simulink model "Series_R2015b"  (R2017a)
settings: Solver=ode4  StartTime=0  StopTime=1200  FixedStep=0.1  MaxStep=0.05  RelTol=1e-5
values from neighbouring files (symbols this model uses):
  Av = 1.725*1.490    (= 2.57025)    [Series_initiate.m]
  Cd = 0.26    [Series_initiate.m]
  Cr = 0.008    [Series_initiate.m]
  Density = (85*19.6e6 + 15*32e6)/100    (= 21460000)    [Series_initiate.m]
  EtaPE = 0.98    [Series_initiate.m]
  gr2 = 5    [Series_initiate.m]
  grav = 9.81    [Series_initiate.m]
  Jgenset = 0.1    [Series_initiate.m]
  kgenset = Jgenset/4/0.05    (= 0.5)    [Series_initiate.m]
  ksoc = Wbatt/400/Tau_charge    (= 11700)    [Series_initiate.m]
  Mv = 1325 + 250    (= 1575)    [Series_initiate.m]
  OnOffMax = SOC_batt_ref_value-eps    [Series_initiate.m]
  OnOffMin = 30    [Series_initiate.m]
  Paux = 600    [Series_initiate.m]
  Pice_max = 20E3    (= 20000)    [Series_initiate.m]
  rho_air = 1.225    [Series_initiate.m]
  rw = 0.30    (= 0.3)    [Series_initiate.m]
  SOC_batt_ref_value = 70    [Series_initiate.m]
  Tau_charge = 1    [Series_initiate.m]
  Tem1_max = 1.2*Tice_max    [Series_initiate.m]
  Tem2_max = 400+105    (= 505)    [Series_initiate.m]
  Tice_max = Pice_max/(wice_max*row/(length(EtaICE)-1))    [Series_initiate.m]
  Wbatt = 100*3600*13    (= 4680000)    [Series_initiate.m]
  wice_max = 4500*2*pi/60    (= 471.238898038)    [Series_initiate.m]
  wice_min = 800*2*pi/60    (= 83.7758040957)    [Series_initiate.m]
undefined symbols (not defined in the file or in its folder): EtaBATT, EtaEM1, EtaEM2, Pbatt, Pice_max_parallel, PtoT, sfunxy, Tlim_ice, Wice
undefined symbols (not defined in the file): EtaICE, FuelConsICE, Pem1_max, Pem2_max, Tem1, Tem2, Tice, Wem1, Wem2
settings Model: ExtModeTrigMode=oneshot  ExtModeArmWhenConnect=off  Creator=matsl  LastModifiedBy=Oskar
settings DataIOCC: SaveFormat=Array  SignalLoggingSaveFormat=ModelDataLogs  SignalLoggingName=sigsOut
settings OptimizationCC: BlockReduction=off  BooleanDataType=off  ExpressionDepthLimit=2147483647  InitFltsAndDblsToZero=on  LifeSpan=inf
settings DebuggingCC: ConsistencyChecking=warning  SaveWithParameterizedLinksMsg=none  UnderspecifiedInitializationDetection=Classic  MergeDetectMultiDrivingBlocksExec=none  SignalResolutionControl=TryResolveAllWithWarning  MultiTaskDSMMsg=warning  MultiTaskCondExecSysMsg=none  UnnecessaryDatatypeConvMsg=warning  FcnCallInpInsideContextMsg=warning  UnconnectedInputMsg=none  UnconnectedOutputMsg=none  UnconnectedLineMsg=none  AllowSymbolicDim=off  StateNameClashWarn=warning  SFUnexpectedBacktrackingDiag=warning  SFNoUnconditionalDefaultTransitionDiag=warning  SFExecutionAtInitializationDiag=none
settings HardwareCC: ProdBitPerPointer=32  ProdBitPerSizeT=32  ProdBitPerPtrDiffT=32  ProdLargestAtomicFloat=None  ProdIntDivRoundTo=Undefined  ProdEndianess=Unspecified  ProdWordSize=32  ProdHWDeviceType=32-bit Generic  TargetUnknown=on
settings ModelReferenceCC: PropagateSignalLabelsOutOfModel=off
settings GRTTargetCC: TargetLangStandard=C89/C90 (ANSI)  CombineOutputUpdateFcns=off  GRTInterface=on
settings ConfigComp: CovMetricSettings=dw  CovHtmlReporting=on  CovSaveCumulativeToWorkspaceVar=on  CovSaveSingleToWorkspaceVar=on  CovExternalEMLEnable=off

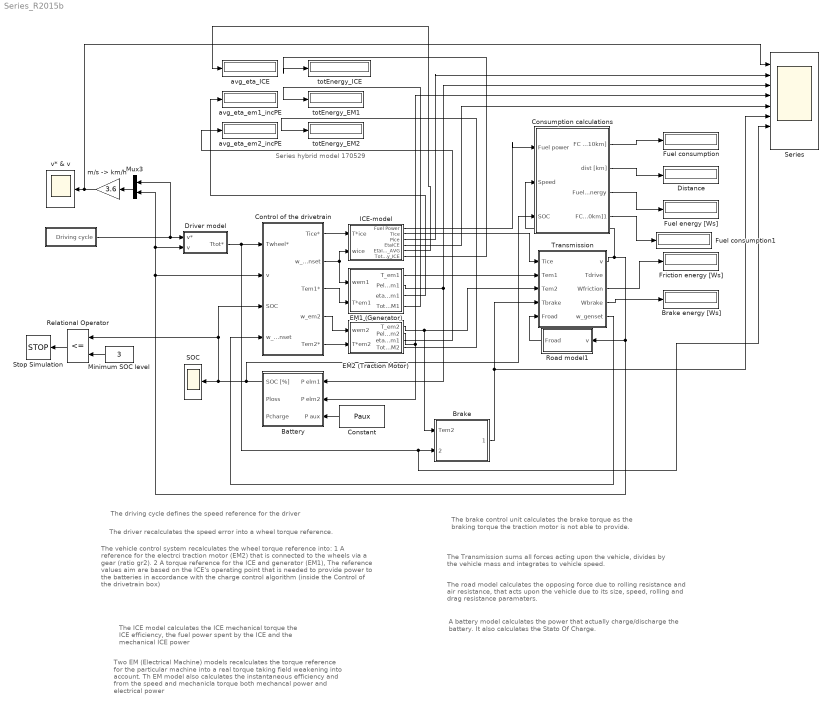
== system Series_R2015b ==
  note: Series hybrid model 170529
  note: The ICE model calculates the ICE mechanical torque
      | the ICE efficiency, the fuel power spent by the ICE
      | and the mechanical ICE power
  note: Two EM (Electrical Machine) models recalculates the
      | torque reference for the particular machine into a real
      | torque taking field weakening into account. Th EM model also
      | calculates the instantaneous efficiency and from the speed
      | and mechanicla torque both mechancal power and electrical power
  note: A battery model calculates the power that actually charge/discharge
      | the battery.
      | It also calculates the Stato Of Charge.
  note: The driving cycle defines the speed reference for the driver
  note: The brake control unit calculates the brake torque as
      | the braking torque the traction motor is not able
      | to provide.
  note: The Transmission sums all forces acting upon the vehicle, divides
      | by the vehicle mass and integrates to vehicle speed.
  note: The road model calculates the opposing force due to rolling resistance
      | and air resistance, that acts upon the vehicle due to its size, speed,
      | rolling and drag resistance paramaters.
  note: The driver recalculates the speed error into a wheel torque reference.
  note: The vehicle control system recalculates the wheel torque reference into:
      | 1	     A reference for the electrci traction motor (EM2) that is
      | connected to the wheels via a gear (ratio gr2).
      | 2	     A torque reference for the ICE and generator (EM1),
      | The reference values aim are based on the ICE's operating point that is needed
      | to provide power to the batteries in accordance with the charge control
      | algorithm (inside the Control of the drivetrain box)
  " " : Subsystem  mask{Cycle=IdealMotion}
      mask prompts: Cycle "Driving cycle"
      mask TypeOptions Cycle: nedc | us06 | IdealMotion
  Battery : Subsystem
  Brake : Subsystem
  Brake energy [Ws] : Display
  Constant : Constant  Value=Paux
  Consumption calculations : Subsystem
  Control of the drivetrain : Subsystem
  Distance : Display
  "Driver model " : Subsystem  mask{Mv=Mv, rw=rw, T_max=Tem2_max*gr2}
      mask prompts: Mv "Vehicle Mass"; rw "Wheel Radius"; T_max "Max Wheel Torque"
      mask init:
      | Ti = 3 + 7*(Mv-1000)/9000;
      | Kv=4*Mv/Ti;
  EM1 (Generator) : Subsystem
  EM2 (Traction Motor) : Subsystem
  Friction energy [Ws] : Display
  Fuel consumption : Display
  Fuel consumption1 : Display
  Fuel energy [Ws] : Display
  ICE-model : Subsystem
  Minimum SOC level : Constant  Value=3
  Mux3 : Mux  Inputs=2
  Relational Operator : RelationalOperator  Operator=<=  OutDataTypeStr=boolean  RndMeth=Nearest
  Road model1 : Subsystem
  SOC : Scope
  Series : Scope  NumInputPorts=8
  Stop Simulation : Stop
  Transmission : Subsystem
  avg_eta_ICE : Display
  avg_eta_em1_incPE : Display
  avg_eta_em2_incPE : Display
  "m/s -> km/h" : Gain  Gain=3.6  SaturateOnIntegerOverflow=on  OutDataTypeStr=Inherit: Same as input  ParamDataTypeStr=Inherit: Same as input
  totEnergy_EM1 : Display
  totEnergy_EM2 : Display
  totEnergy_ICE : Display
  v* & v : Scope
  wires:
  Constant/1 -> Battery/3(P aux)
  " "/1(Driving cycle) -> Mux3/1, "Driver model "/1(v*)
  "Driver model "/1(Ttot*) -> Series/7, Brake/2(T*wheel), Control of the drivetrain/1(Twheel*)
  Mux3/1 -> "m/s -> km/h"/1
  Transmission/1(v) -> Consumption calculations/2(Speed), Control of the drivetrain/2(v), Mux3/2, "Driver model "/2(v), Road model1/1("v ")
  ICE-model/1(Fuel Power) -> Consumption calculations/1(Fuel power)
  Transmission/3(Wfriction) -> Friction energy [Ws]/1
  Transmission/4(Wbrake) -> Brake energy [Ws]/1
  Brake/1(T_brake) -> Transmission/4(Tbrake), Series/6
  ICE-model/2(Tice) -> Transmission/1(Tice)
  EM1 (Generator)/1(T_em1) -> Transmission/2(Tem1)
  EM2 (Traction Motor)/1(T_em2) -> Brake/1(Tem2), Transmission/3(Tem2)
  Control of the drivetrain/3(Tem1*) -> EM1 (Generator)/2(T*em1)
  Control of the drivetrain/1(Tice*) -> ICE-model/1(T*ice)
  Control of the drivetrain/2("w_genset ") -> EM1 (Generator)/1(wem1), ICE-model/2(wice)
  Transmission/5(w_genset) -> Control of the drivetrain/4(w_genset)
  Control of the drivetrain/4(w_em2) -> EM2 (Traction Motor)/1(wem2)
  EM1 (Generator)/2(Pel_em1) -> Battery/1(P elm1), Series/3
  EM2 (Traction Motor)/2(Pel_em2) -> Battery/2(P elm2), Series/4
  ICE-model/3(Pice) -> Series/2
  ICE-model/4(EtaICE) -> Series/5
  Control of the drivetrain/5(Tem2*) -> EM2 (Traction Motor)/2(T*em2)
  Consumption calculations/1(FC [l/10km]) -> Fuel consumption/1
  Consumption calculations/3(FuelEnergy) -> Fuel energy [Ws]/1
  Road model1/1(Froad) -> Transmission/5(Froad)
  "m/s -> km/h"/1 -> Series/1, v* & v/1
  Consumption calculations/2(dist [km]) -> Distance/1
  Relational Operator/1 -> Stop Simulation/1
  Minimum SOC level/1 -> Relational Operator/2
  Battery/1(SOC [%]) -> Consumption calculations/3(SOC), Relational Operator/1, Control of the drivetrain/3(SOC), SOC/1
  EM1 (Generator)/3(eta_avg_em1) -> avg_eta_em1_incPE/1
  EM2 (Traction Motor)/3(eta_avg_em1) -> avg_eta_em2_incPE/1
  ICE-model/5(EtaICE_AVG) -> avg_eta_ICE/1
  EM2 (Traction Motor)/4(Total_Energy_EM2) -> totEnergy_EM2/1
  EM1 (Generator)/4(Total_Energy_EM1) -> totEnergy_EM1/1
  ICE-model/6(Total_Energy_ICE) -> totEnergy_ICE/1
  Consumption calculations/4(FC_TOT [l/10km]1) -> Fuel consumption1/1

== system Series_R2015b/  ==
  Constant : Constant  Value=Cycle
  Multiport Switch : MultiPortSwitch  SaturateOnIntegerOverflow=on  InputSameDT=on
  v-buss1 : FromWorkspace  VariableName=us06  SampleTime=.1
  v-buss2 : FromWorkspace  VariableName=IdealMotion  SampleTime=.1
  v-buss8 : FromWorkspace  VariableName=nedc  SampleTime=.1
  Driving cycle : Outport
  wires:
  v-buss8/1 -> Multiport Switch/2
  Constant/1 -> Multiport Switch/1
  v-buss1/1 -> Multiport Switch/3
  v-buss2/1 -> Multiport Switch/4
  Multiport Switch/1 -> Driving cycle/1

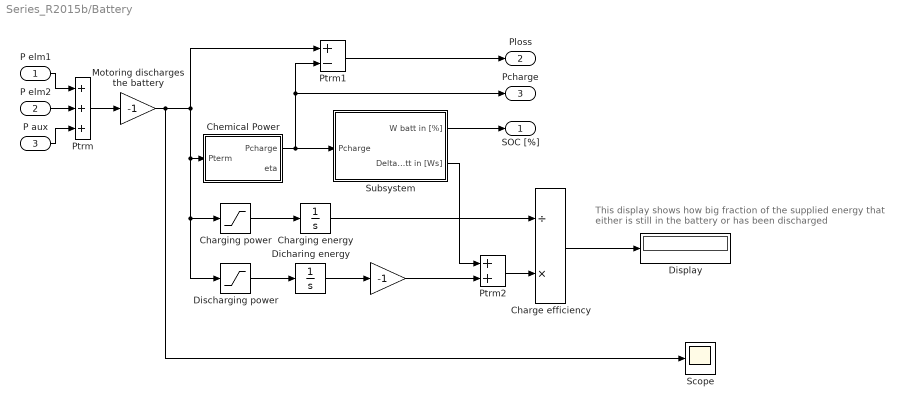
== system Series_R2015b/Battery ==
  note: This display shows how big fraction of the supplied energy
      | that either is still in the battery or has been discharged
  P elm1 : Inport
  P elm2 : Inport  Port=2
  P aux : Inport  Port=3
  " " : Gain  Gain=-1  SaturateOnIntegerOverflow=on  OutDataTypeStr=Inherit: Same as input  ParamDataTypeStr=Inherit: Same as input
  Charge efficiency : Product  Inputs=/*  SaturateOnIntegerOverflow=on  OutDataTypeStr=Inherit: Same as first input
  Charging energy : Integrator  InitialCondition=1  LimitOutput=on  LowerSaturationLimit=1
  Charging power : Saturate  UpperLimit=inf  LowerLimit=0
  Chemical Power : Subsystem
  Dicharing energy : Integrator  InitialCondition=-1  LimitOutput=on  UpperSaturationLimit=-1
  Discharging power : Saturate  UpperLimit=0  LowerLimit=-inf
  Display : Display
  Motoring discharges the battery : Gain  Gain=-1  SaturateOnIntegerOverflow=on  OutDataTypeStr=Inherit: Same as input  ParamDataTypeStr=Inherit: Same as input
  Ptrm : Sum  Inputs=+++  SaturateOnIntegerOverflow=on  InputSameDT=on  OutDataTypeStr=Inherit: Same as first input
  Ptrm1 : Sum  Inputs=+-  SaturateOnIntegerOverflow=on  InputSameDT=on  OutDataTypeStr=Inherit: Same as first input
  Ptrm2 : Sum  SaturateOnIntegerOverflow=on  InputSameDT=on  OutDataTypeStr=Inherit: Same as first input
  Scope : Scope
  Subsystem : Subsystem
  SOC [%] : Outport  InitialOutput=0
  Ploss : Outport  Port=2  InitialOutput=0
  Pcharge : Outport  Port=3  InitialOutput=0
  wires:
  P elm1/1 -> Ptrm/1
  Ptrm/1 -> Motoring discharges the battery/1
  Subsystem/1(W batt in [%]) -> SOC [%]/1
  P aux/1 -> Ptrm/3
  P elm2/1 -> Ptrm/2
  Chemical Power/1(Pcharge) -> Ptrm1/2, Pcharge/1, Subsystem/1("Pcharge ")
  Ptrm1/1 -> Ploss/1
  Motoring discharges the battery/1 -> Ptrm1/1, Charging power/1, Discharging power/1, Chemical Power/1(Pterm), Scope/1
  Charge efficiency/1 -> Display/1
  Charging power/1 -> Charging energy/1
  Discharging power/1 -> Dicharing energy/1
  Dicharing energy/1 -> " "/1
  Subsystem/2(DeltaWbatt in [Ws]) -> Ptrm2/1
  " "/1 -> Ptrm2/2
  Ptrm2/1 -> Charge efficiency/2
  Charging energy/1 -> Charge efficiency/1

== system Series_R2015b/Brake ==
  note: The mechanical brake is used when the traction motor is
      | not strong enough.
  Tem2 : Inport
  T*wheel : Inport  Port=2
  Brake : Scope  NumInputPorts=3
  Final gear : Gain  Gain=gr2  SaturateOnIntegerOverflow=on  OutDataTypeStr=Inherit: Same as input  ParamDataTypeStr=Inherit: Same as input
  Only negative brake torque : Saturate  UpperLimit=0  LowerLimit=-inf
  Sum3 : Sum  Inputs=+-  SaturateOnIntegerOverflow=on  InputSameDT=on  OutDataTypeStr=Inherit: Same as first input
  T_brake : Outport  InitialOutput=0
  wires:
  Sum3/1 -> Only negative brake torque/1
  Only negative brake torque/1 -> Brake/3, T_brake/1
  Tem2/1 -> Final gear/1
  T*wheel/1 -> Brake/1, Sum3/1
  Final gear/1 -> Brake/2, Sum3/2

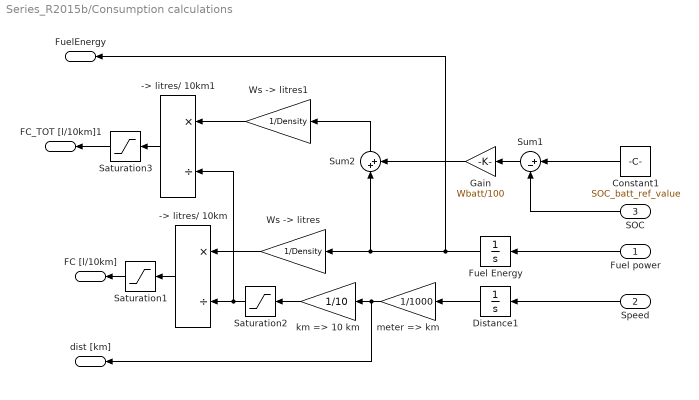
== system Series_R2015b/Consumption calculations ==
  Fuel power : Inport
  Speed : Inport  Port=2
  SOC : Inport  Port=3
  -> litres/ 10km : Product  Inputs=*/  SaturateOnIntegerOverflow=on  InputSameDT=on  OutDataTypeStr=Inherit: Same as first input
  -> litres/ 10km1 : Product  Inputs=*/  SaturateOnIntegerOverflow=on  InputSameDT=on  OutDataTypeStr=Inherit: Same as first input
  Constant1 : Constant  Value=SOC_batt_ref_value
  Distance1 : Integrator
  Fuel Energy : Integrator
  Gain : Gain  Gain=Wbatt/100
  Saturation1 : Saturate  UpperLimit=5  LowerLimit=eps
  Saturation2 : Saturate  UpperLimit=inf  LowerLimit=eps
  Saturation3 : Saturate  UpperLimit=5  LowerLimit=eps
  Sum1 : Sum  Inputs=|+-
  Sum2 : Sum  Inputs=|++
  "Ws -> litres" : Gain  Gain=1/Density  SaturateOnIntegerOverflow=on  OutDataTypeStr=Inherit: Same as input  ParamDataTypeStr=Inherit: Same as input
  "Ws -> litres1" : Gain  Gain=1/Density  SaturateOnIntegerOverflow=on  OutDataTypeStr=Inherit: Same as input  ParamDataTypeStr=Inherit: Same as input
  km => 10 km : Gain  Gain=1/10  SaturateOnIntegerOverflow=on  OutDataTypeStr=Inherit: Same as input  ParamDataTypeStr=Inherit: Same as input
  meter => km : Gain  Gain=1/1000  SaturateOnIntegerOverflow=on  OutDataTypeStr=Inherit: Same as input  ParamDataTypeStr=Inherit: Same as input
  FC [l/10km] : Outport
  dist [km] : Outport  Port=2
  FuelEnergy : Outport  Port=3
  FC_TOT [l/10km]1 : Outport  Port=4
  wires:
  Fuel power/1 -> Fuel Energy/1
  Fuel Energy/1 -> FuelEnergy/1, Sum2/1, "Ws -> litres"/1
  meter => km/1 -> dist [km]/1, km => 10 km/1
  Speed/1 -> Distance1/1
  -> litres/ 10km/1 -> Saturation1/1
  Distance1/1 -> meter => km/1
  "Ws -> litres"/1 -> -> litres/ 10km/1
  Saturation1/1 -> FC [l/10km]/1
  km => 10 km/1 -> Saturation2/1
  Saturation2/1 -> -> litres/ 10km1/2, -> litres/ 10km/2
  -> litres/ 10km1/1 -> Saturation3/1
  Saturation3/1 -> FC_TOT [l/10km]1/1
  "Ws -> litres1"/1 -> -> litres/ 10km1/1
  Constant1/1 -> Sum1/1
  Sum2/1 -> "Ws -> litres1"/1
  Gain/1 -> Sum2/2
  Sum1/1 -> Gain/1
  SOC/1 -> Sum1/2

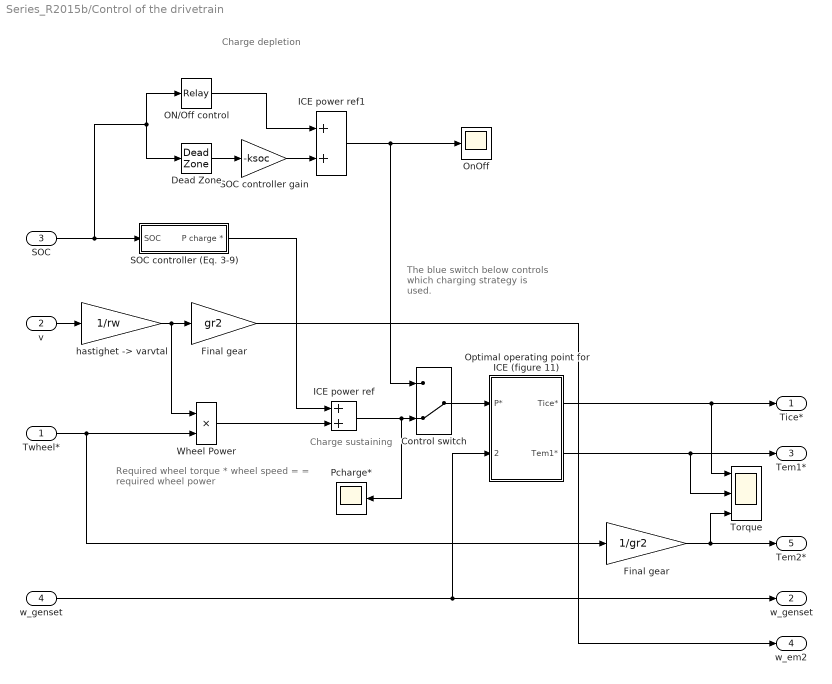
== system Series_R2015b/Control of the drivetrain ==
  note: The blue switch below
      | controls which charging
      | strategy is used.
  note: Required wheel torque * wheel speed =
      | = required wheel power
  note: Charge depletion
  note: Charge sustaining
  Twheel* : Inport
  v : Inport  Port=2
  SOC : Inport  Port=3
  w_genset : Inport  Port=4
  Control switch : ManualSwitch  CurrentSetting=0
  Dead Zone : DeadZone  LowerValue=OnOffMin  UpperValue=OnOffMax  SaturateOnIntegerOverflow=on
  Final gear : Gain  Gain=1/gr2  SaturateOnIntegerOverflow=on  OutDataTypeStr=Inherit: Same as input  ParamDataTypeStr=Inherit: Same as input
  "Final gear " : Gain  Gain=gr2  SaturateOnIntegerOverflow=on  OutDataTypeStr=Inherit: Same as input  ParamDataTypeStr=Inherit: Same as input
  ICE power ref : Sum  SaturateOnIntegerOverflow=on  InputSameDT=on  OutDataTypeStr=Inherit: Same as first input
  ICE power ref1 : Sum  SaturateOnIntegerOverflow=on  InputSameDT=on  OutDataTypeStr=Inherit: Same as first input
  ON/Off control : Relay  OnSwitchValue=OnOffMax  OffSwitchValue=OnOffMin  OnOutputValue=0  OffOutputValue=ksoc
  OnOff : Scope
  Optimal operating point for ICE (figure 11) : Subsystem
  Pcharge* : Scope
  SOC controller (Eq. 3-9) : Subsystem
  SOC controller gain : Gain  Gain=-ksoc  OutDataTypeStr=Inherit: Same as input  ParamDataTypeStr=Inherit: Same as input
  Torque : Scope  NumInputPorts=3
  Wheel Power : Product  SaturateOnIntegerOverflow=on  InputSameDT=on  OutDataTypeStr=Inherit: Same as first input
  "hastighet -> varvtal" : Gain  Gain=1/rw  SaturateOnIntegerOverflow=on  OutDataTypeStr=Inherit: Same as input  ParamDataTypeStr=Inherit: Same as input
  Tice* : Outport
  "w_genset " : Outport  Port=2
  Tem1* : Outport  Port=3
  w_em2 : Outport  Port=4
  Tem2* : Outport  Port=5
  wires:
  "hastighet -> varvtal"/1 -> Wheel Power/1, "Final gear "/1
  Twheel*/1 -> Wheel Power/2, Final gear/1
  v/1 -> "hastighet -> varvtal"/1
  SOC/1 -> SOC controller (Eq. 3-9)/1(SOC), Dead Zone/1, ON/Off control/1
  Wheel Power/1 -> ICE power ref/2
  SOC controller (Eq. 3-9)/1(P charge *) -> ICE power ref/1
  Optimal operating point for ICE (figure 11)/2(Tem1*) -> Tem1*/1, Torque/2
  Optimal operating point for ICE (figure 11)/1(Tice*) -> Tice*/1, Torque/1
  w_genset/1 -> Optimal operating point for ICE (figure 11)/2(w_genset), "w_genset "/1
  Final gear/1 -> Tem2*/1, Torque/3
  "Final gear "/1 -> w_em2/1
  Dead Zone/1 -> SOC controller gain/1
  ON/Off control/1 -> ICE power ref1/1
  SOC controller gain/1 -> ICE power ref1/2
  Control switch/1 -> Optimal operating point for ICE (figure 11)/1(P*)
  ICE power ref1/1 -> OnOff/1, Control switch/1
  ICE power ref/1 -> Control switch/2, Pcharge*/1

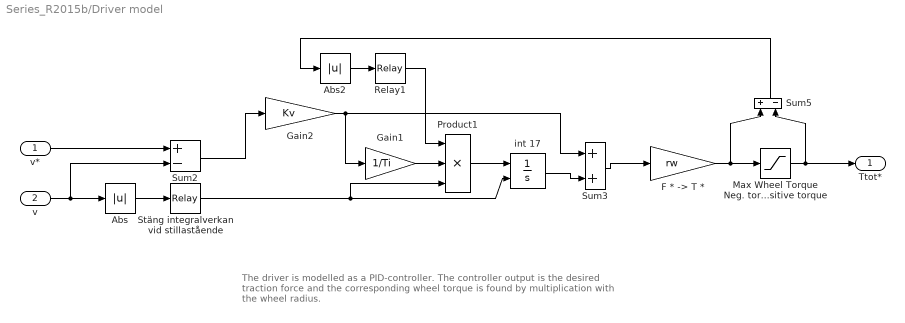
== system Series_R2015b/Driver model  ==
  note: The driver is modelled as a PID-controller.
      | The controller output is the desired traction force and the
      | corresponding wheel torque is found by multiplication with the wheel radius.
  v* : Inport
  v : Inport  Port=2
  Abs : Abs  SaturateOnIntegerOverflow=on
  Abs2 : Abs  SaturateOnIntegerOverflow=on
  "F * -> T *" : Gain  Gain=rw  SaturateOnIntegerOverflow=on  OutDataTypeStr=Inherit: Same as input  ParamDataTypeStr=Inherit: Same as input
  Gain1 : Gain  Gain=1/Ti  SaturateOnIntegerOverflow=on  OutDataTypeStr=Inherit: Same as input  ParamDataTypeStr=Inherit: Same as input
  Gain2 : Gain  Gain=Kv  SaturateOnIntegerOverflow=on  OutDataTypeStr=Inherit: Same as input  ParamDataTypeStr=Inherit: Same as input
  Max Wheel Torque Neg. torque can be 5 times positive torque : Saturate  UpperLimit=T_max  LowerLimit=-T_max*5
  Product1 : Product  Inputs=3  SaturateOnIntegerOverflow=on  InputSameDT=on  OutDataTypeStr=Inherit: Same as first input
  Relay1 : Relay  OnOutputValue=0  OffOutputValue=1
  Stäng integralverkan vid stillastående : Relay  OnSwitchValue=0.3  OffSwitchValue=0.3-eps
  Sum2 : Sum  Inputs=+-  SaturateOnIntegerOverflow=on  InputSameDT=on  OutDataTypeStr=Inherit: Same as first input
  Sum3 : Sum  SaturateOnIntegerOverflow=on  InputSameDT=on  OutDataTypeStr=Inherit: Same as first input
  Sum5 : Sum  Inputs=+-  SaturateOnIntegerOverflow=on  InputSameDT=on  OutDataTypeStr=Inherit: Same as first input
  int 17 : Integrator  ExternalReset=falling  LimitOutput=on  UpperSaturationLimit=1000  LowerSaturationLimit=-10000
  Ttot* : Outport  InitialOutput=0
  wires:
  v/1 -> Sum2/2, Abs/1
  v*/1 -> Sum2/1
  Sum2/1 -> Gain2/1
  Stäng integralverkan vid stillastående/1 -> int 17/2, Product1/3
  Gain2/1 -> Sum3/1, Gain1/1
  "F * -> T *"/1 -> Max Wheel Torque Neg. torque can be 5 times positive torque/1, Sum5/1
  int 17/1 -> Sum3/2
  Sum3/1 -> "F * -> T *"/1
  Product1/1 -> int 17/1
  Abs/1 -> Stäng integralverkan vid stillastående/1
  Gain1/1 -> Product1/2
  Abs2/1 -> Relay1/1
  Relay1/1 -> Product1/1
  Sum5/1 -> Abs2/1
  Max Wheel Torque Neg. torque can be 5 times positive torque/1 -> Ttot*/1, Sum5/2

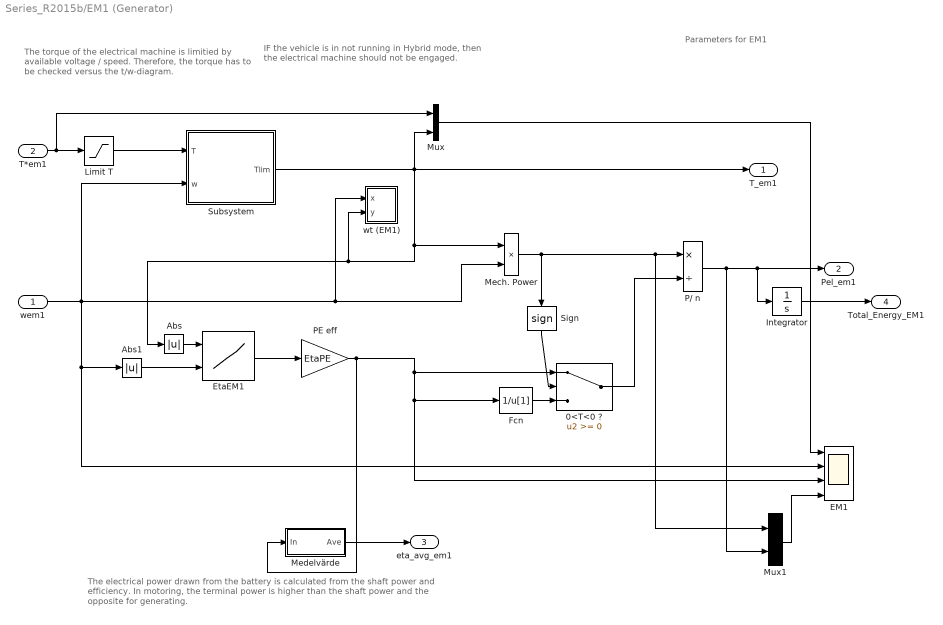
== system Series_R2015b/EM1 (Generator) ==
  note: The torque of the electrical machine is
      | limitied by available voltage / speed. Therefore, the
      | torque has to be checked versus the t/w-diagram.
  note: IF the vehicle is in not running in Hybrid mode, then
      | the electrical machine should not be engaged.
  note: The electrical power drawn from the battery is calculated from the shaft power and
      | efficiency. In motoring, the terminal power is higher than the shaft power and
      | the opposite for  generating.
  note: Parameters for EM1
  wem1 : Inport
  T*em1 : Inport  Port=2
  0<T<0 ? : Switch  SaturateOnIntegerOverflow=on  InputSameDT=on
  Abs : Abs  SaturateOnIntegerOverflow=on
  Abs1 : Abs  SaturateOnIntegerOverflow=on
  EM1 : Scope  NumInputPorts=4
  EtaEM1 : Lookup2D  RowIndex=Tem1  ColumnIndex=Wem1  Table=EtaEM1  LookUpMeth=Interpolation-Use End Values  SaturateOnIntegerOverflow=on
  Fcn : Fcn  Expr=1/u[1]
  Integrator : Integrator
  Limit T : Saturate  UpperLimit=Tem1_max  LowerLimit=-Tem1_max
  Mech. Power : Product  SaturateOnIntegerOverflow=on  OutDataTypeStr=Inherit: Same as first input
  Medelvärde : Subsystem
  Mux : Mux  Inputs=2
  Mux1 : Mux  Inputs=2
  P/ n : Product  Inputs=*/  SaturateOnIntegerOverflow=on  InputSameDT=on  OutDataTypeStr=Inherit: Same as first input
  PE eff : Gain  Gain=EtaPE  SaturateOnIntegerOverflow=on  OutDataTypeStr=Inherit: Same as input  ParamDataTypeStr=Inherit: Same as input
  Sign : Signum
  Subsystem : Subsystem  mask{Tmax=Tem1_max, Pmax=Pem1_max}
      mask prompts: Tmax "Max Torque"; Pmax "Max Power"
      mask Display:
      | plot(-120,-120,120,120)
      | plot([-110 110],[0 0],[0 0],[-110 110])
      | plot([-20 20],[90 90],[-20 20],[-90 -90])
      | 
      | plot([-100 :-20],-90*20./[-100:-20])
      | plot([-100 :-20],90*20./[-100:-20])
      | plot([20:100],-90*20./[20:100])
      | plot([20:100],90*20./[20:100])
  wt (EM1) : Subsystem  AncestorBlock=simulink/Sinks/XY Graph  LoadFcn=sfunxy([],[],[],'LoadBlock')  StartFcn=sfunxy([],[],[],'Start')  StopFcn=sfunxy([],[],[],'Stop')  TreatAsAtomicUnit=on  SimViewingDevice=on  mask(XY scope.){xmin=-max(Wem1)*1.2, xmax=max(Wem1)*1.2, ymin=-max(Tem1)*1.2, ymax=max(Tem1)*1.2, st=1}
      mask prompts: xmin "x-min:"; xmax "x-max:"; ymin "y-min:"; ymax "y-max:"; st "Sample time:"
      mask help: Plots second input (Y) against first input (X) at each time step to create an X-Y plot. Ignores data outside the ranges specified by x-min, x-max, y-min, y-max.
      settings: CopyFcn=sfunxy([],[],[],'CopyBlock')  DeleteFcn=sfunxy([],[],[],'DeleteBlock')  NameChangeFcn=sfunxy([],[],[],'NameChange')
      mask Help: This block can be used to explore limit cycles. Look at the m-file sfunxy.m to see how it works.
      mask Display: plot([.05 .95 .95 .05 .05],[.45 .45 .95 .95 .45], 0.5+cos(0:0.1:2*pi)*0.3,0.7+sin(0:0.1:2*pi)*0.2)
  T_em1 : Outport  InitialOutput=0
  Pel_em1 : Outport  Port=2  InitialOutput=0
  eta_avg_em1 : Outport  Port=3  InitialOutput=0
  Total_Energy_EM1 : Outport  Port=4  InitialOutput=0
  wires:
  EtaEM1/1 -> PE eff/1
  Subsystem/1(Tlim) -> Mech. Power/1, wt (EM1)/2(y), Abs/1, T_em1/1, Mux/2
  Sign/1 -> 0<T<0 ?/2
  P/ n/1 -> Mux1/2, Integrator/1, Pel_em1/1
  T*em1/1 -> Limit T/1, Mux/1
  Fcn/1 -> 0<T<0 ?/3
  0<T<0 ?/1 -> P/ n/2
  Abs/1 -> EtaEM1/1
  Limit T/1 -> Subsystem/1(T)
  wem1/1 -> EM1/2, Abs1/1, wt (EM1)/1(x), Mech. Power/2, Subsystem/2(w)
  PE eff/1 -> Medelvärde/1(In), EM1/3, Fcn/1, 0<T<0 ?/1
  Mux/1 -> EM1/1
  Mux1/1 -> EM1/4
  Mech. Power/1 -> Sign/1, Mux1/1, P/ n/1
  Abs1/1 -> EtaEM1/2
  Medelvärde/1(Ave) -> eta_avg_em1/1
  Integrator/1 -> Total_Energy_EM1/1

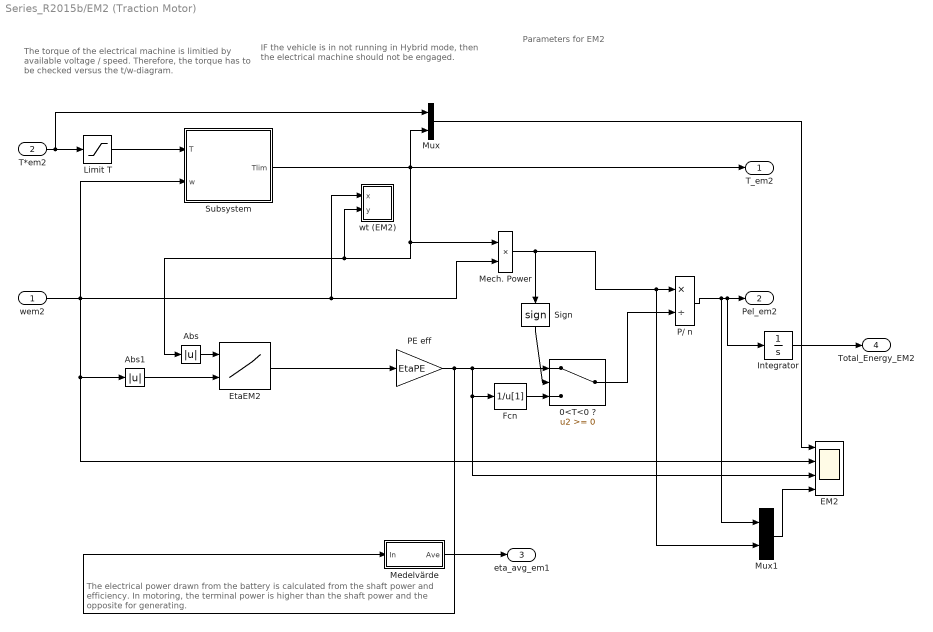
== system Series_R2015b/EM2 (Traction Motor) ==
  note: The torque of the electrical machine is
      | limitied by available voltage / speed. Therefore, the
      | torque has to be checked versus the t/w-diagram.
  note: IF the vehicle is in not running in Hybrid mode, then
      | the electrical machine should not be engaged.
  note: The electrical power drawn from the battery is calculated from the shaft power and
      | efficiency. In motoring, the terminal power is higher than the shaft power and
      | the opposite for  generating.
  note: Parameters for EM2
  wem2 : Inport
  T*em2 : Inport  Port=2
  0<T<0 ? : Switch  SaturateOnIntegerOverflow=on  InputSameDT=on
  Abs : Abs  SaturateOnIntegerOverflow=on
  Abs1 : Abs  SaturateOnIntegerOverflow=on
  EM2 : Scope  NumInputPorts=4
  EtaEM2 : Lookup2D  RowIndex=Tem2  ColumnIndex=Wem2  Table=EtaEM2  LookUpMeth=Interpolation-Use End Values  SaturateOnIntegerOverflow=on
  Fcn : Fcn  Expr=1/u[1]
  Integrator : Integrator
  Limit T : Saturate  UpperLimit=Tem2_max  LowerLimit=-Tem2_max
  Mech. Power : Product  SaturateOnIntegerOverflow=on  OutDataTypeStr=Inherit: Same as first input
  Medelvärde : Subsystem
  Mux : Mux  Inputs=2
  Mux1 : Mux  Inputs=2
  P/ n : Product  Inputs=*/  SaturateOnIntegerOverflow=on  InputSameDT=on  OutDataTypeStr=Inherit: Same as first input
  PE eff : Gain  Gain=EtaPE  SaturateOnIntegerOverflow=on  OutDataTypeStr=Inherit: Same as input  ParamDataTypeStr=Inherit: Same as input
  Sign : Signum
  Subsystem : Subsystem  mask{Tmax=Tem2_max, Pmax=Pem2_max}
      mask prompts: Tmax "Max Torque"; Pmax "Max Power"
      mask Display:
      | plot(-120,-120,120,120)
      | plot([-110 110],[0 0],[0 0],[-110 110])
      | plot([-20 20],[90 90],[-20 20],[-90 -90])
      | 
      | plot([-100 :-20],-90*20./[-100:-20])
      | plot([-100 :-20],90*20./[-100:-20])
      | plot([20:100],-90*20./[20:100])
      | plot([20:100],90*20./[20:100])
  wt (EM2) : Subsystem  AncestorBlock=simulink/Sinks/XY Graph  LoadFcn=sfunxy([],[],[],'LoadBlock')  StartFcn=sfunxy([],[],[],'Start')  StopFcn=sfunxy([],[],[],'Stop')  TreatAsAtomicUnit=on  SimViewingDevice=on  mask(XY scope.){xmin=-max(Wem2)*1.2, xmax=max(Wem2)*1.2, ymin=-max(Tem2)*1.2, ymax=max(Tem2)*1.2, st=1}
      mask prompts: xmin "x-min:"; xmax "x-max:"; ymin "y-min:"; ymax "y-max:"; st "Sample time:"
      mask help: Plots second input (Y) against first input (X) at each time step to create an X-Y plot. Ignores data outside the ranges specified by x-min, x-max, y-min, y-max.
      settings: CopyFcn=sfunxy([],[],[],'CopyBlock')  DeleteFcn=sfunxy([],[],[],'DeleteBlock')  NameChangeFcn=sfunxy([],[],[],'NameChange')
      mask Help: This block can be used to explore limit cycles. Look at the m-file sfunxy.m to see how it works.
      mask Display: plot([.05 .95 .95 .05 .05],[.45 .45 .95 .95 .45], 0.5+cos(0:0.1:2*pi)*0.3,0.7+sin(0:0.1:2*pi)*0.2)
  T_em2 : Outport  InitialOutput=0
  Pel_em2 : Outport  Port=2  InitialOutput=0
  eta_avg_em1 : Outport  Port=3  InitialOutput=0
  Total_Energy_EM2 : Outport  Port=4  InitialOutput=0
  wires:
  EtaEM2/1 -> PE eff/1
  Subsystem/1(Tlim) -> Mech. Power/1, wt (EM2)/2(y), Abs/1, T_em2/1, Mux/2
  Sign/1 -> 0<T<0 ?/2
  P/ n/1 -> Mux1/1, Integrator/1, Pel_em2/1
  T*em2/1 -> Limit T/1, Mux/1
  Fcn/1 -> 0<T<0 ?/3
  0<T<0 ?/1 -> P/ n/2
  Abs/1 -> EtaEM2/1
  Limit T/1 -> Subsystem/1(T)
  wem2/1 -> EM2/2, Abs1/1, wt (EM2)/1(x), Mech. Power/2, Subsystem/2(w)
  Mux/1 -> EM2/1
  Mux1/1 -> EM2/4
  Mech. Power/1 -> Sign/1, Mux1/2, P/ n/1
  Abs1/1 -> EtaEM2/2
  PE eff/1 -> Medelvärde/1(In), EM2/3, Fcn/1, 0<T<0 ?/1
  Medelvärde/1(Ave) -> eta_avg_em1/1
  Integrator/1 -> Total_Energy_EM2/1

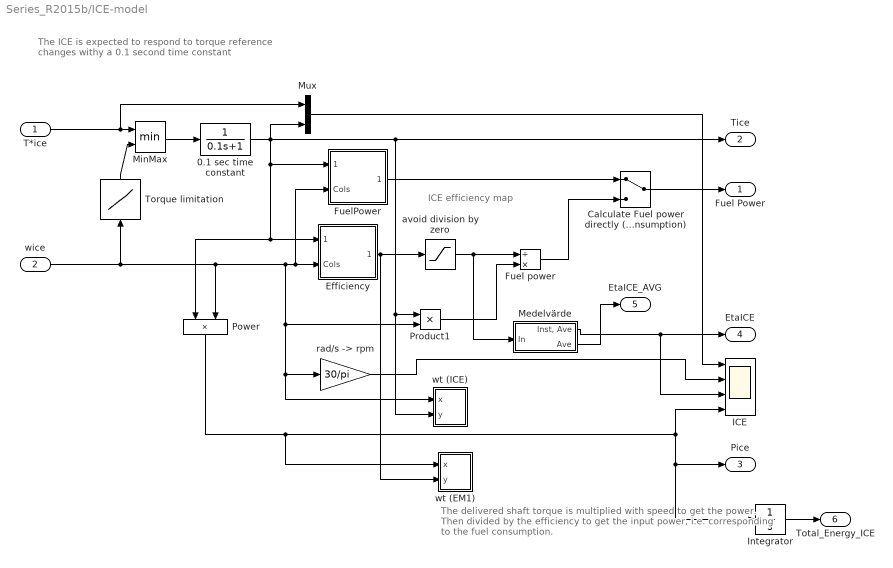
== system Series_R2015b/ICE-model ==
  note: The ICE is expected to respond to torque reference
      | changes withy a 0.1 second
      | time constant
  note: ICE efficiency map
  note: The delivered shaft torque is multiplied with speed to get the power.
      | Then divided by the efficiency to get the input power, i.e.
      | corresponding to the fuel consumption.
  T*ice : Inport
  wice : Inport  Port=2
  0.1 sec time constant : TransferFcn  Denominator=[0.1 1]
  Calculate Fuel power directly (w/o idle consumption) : ManualSwitch
  Efficiency : Subsystem  mask(Lookup Table (2-D)){x=Tice, y=Wice, t=EtaICE}
      mask prompts: x "Row:"; y "Column:"; t "Table:"
      mask help: Performs 2-D linear interpolation of input values using the specified input/output table. Extrapolation is performed outside the table boundaries. The first dimension corresponds to the top (or left) input port.
      mask init:
      | [r,c]=size(t);
      | xt=reshape(x,prod(size(x)),1);
      | xi=xt(:,ones(1,c));
      | minx=min(x); maxx=max(x);
      | mint=min(min(t)); maxt=max(max(t));
      mask Display: plot(double(xi),double(t),double([minx maxx]),double([mint mint]),double([minx minx]),double([mint maxt]))
  Fuel power : Product  Inputs=/*  SaturateOnIntegerOverflow=on  InputSameDT=on  OutDataTypeStr=Inherit: Same as first input
  FuelPower : Subsystem  mask(Lookup Table (2-D)){x=Tice, y=Wice, t=FuelConsICE}
      mask prompts: x "Row:"; y "Column:"; t "Table:"
      mask help: Performs 2-D linear interpolation of input values using the specified input/output table. Extrapolation is performed outside the table boundaries. The first dimension corresponds to the top (or left) input port.
      mask init:
      | [r,c]=size(t);
      | xt=reshape(x,prod(size(x)),1);
      | xi=xt(:,ones(1,c));
      | minx=min(x); maxx=max(x);
      | mint=min(min(t)); maxt=max(max(t));
      mask Display: plot(double(xi),double(t),double([minx maxx]),double([mint mint]),double([minx minx]),double([mint maxt]))
  ICE : Scope  NumInputPorts=4
  Integrator : Integrator
  Medelvärde : Subsystem
  MinMax : MinMax  Inputs=2  SaturateOnIntegerOverflow=on  InputSameDT=on
  Mux : Mux  Inputs=2
  Power : Product  SaturateOnIntegerOverflow=on  OutDataTypeStr=Inherit: Same as first input
  Product1 : Product  SaturateOnIntegerOverflow=on  InputSameDT=on  OutDataTypeStr=Inherit: Same as first input
  Torque limitation : Lookup  InputValues=Wice  Table=Tlim_ice  SaturateOnIntegerOverflow=on
  avoid division by zero : Saturate  UpperLimit=inf  LowerLimit=0.02
  "rad/s -> rpm" : Gain  Gain=30/pi  SaturateOnIntegerOverflow=on  OutDataTypeStr=Inherit: Same as input  ParamDataTypeStr=Inherit: Same as input
  wt (EM1) : Subsystem  AncestorBlock=simulink/Sinks/XY Graph  LoadFcn=sfunxy([],[],[],'LoadBlock')  StartFcn=sfunxy([],[],[],'Start')  StopFcn=sfunxy([],[],[],'Stop')  TreatAsAtomicUnit=on  SimViewingDevice=on  mask(XY scope.){xmin=0, xmax=Pice_max, ymin=0, ymax=1, st=1}
      mask prompts: xmin "x-min:"; xmax "x-max:"; ymin "y-min:"; ymax "y-max:"; st "Sample time:"
      mask help: Plots second input (Y) against first input (X) at each time step to create an X-Y plot. Ignores data outside the ranges specified by x-min, x-max, y-min, y-max.
      settings: CopyFcn=sfunxy([],[],[],'CopyBlock')  DeleteFcn=sfunxy([],[],[],'DeleteBlock')  NameChangeFcn=sfunxy([],[],[],'NameChange')
      mask Help: This block can be used to explore limit cycles. Look at the m-file sfunxy.m to see how it works.
      mask Display: plot([.05 .95 .95 .05 .05],[.45 .45 .95 .95 .45], 0.5+cos(0:0.1:2*pi)*0.3,0.7+sin(0:0.1:2*pi)*0.2)
  wt (ICE) : Subsystem  AncestorBlock=simulink/Sinks/XY Graph  LoadFcn=sfunxy([],[],[],'LoadBlock')  StartFcn=sfunxy([],[],[],'Start')  StopFcn=sfunxy([],[],[],'Stop')  TreatAsAtomicUnit=on  SimViewingDevice=on  mask(XY scope.){xmin=0, xmax=max(Wice)*1.2, ymin=-max(Tice)*0.2, ymax=max(Tice)*1.2, st=1}
      mask prompts: xmin "x-min:"; xmax "x-max:"; ymin "y-min:"; ymax "y-max:"; st "Sample time:"
      mask help: Plots second input (Y) against first input (X) at each time step to create an X-Y plot. Ignores data outside the ranges specified by x-min, x-max, y-min, y-max.
      settings: CopyFcn=sfunxy([],[],[],'CopyBlock')  DeleteFcn=sfunxy([],[],[],'DeleteBlock')  NameChangeFcn=sfunxy([],[],[],'NameChange')
      mask Help: This block can be used to explore limit cycles. Look at the m-file sfunxy.m to see how it works.
      mask Display: plot([.05 .95 .95 .05 .05],[.45 .45 .95 .95 .45], 0.5+cos(0:0.1:2*pi)*0.3,0.7+sin(0:0.1:2*pi)*0.2)
  Fuel Power : Outport  InitialOutput=0
  Tice : Outport  Port=2  InitialOutput=0
  Pice : Outport  Port=3  InitialOutput=0
  EtaICE : Outport  Port=4  InitialOutput=0
  EtaICE_AVG : Outport  Port=5  InitialOutput=0
  Total_Energy_ICE : Outport  Port=6  InitialOutput=0
  wires:
  Product1/1 -> Fuel power/2
  Efficiency/1(Out1) -> wt (EM1)/2(y), avoid division by zero/1
  "rad/s -> rpm"/1 -> ICE/2
  Medelvärde/1("Inst, Ave") -> ICE/3, EtaICE/1
  T*ice/1 -> Mux/1, MinMax/1
  Torque limitation/1 -> MinMax/2
  MinMax/1 -> 0.1 sec time constant/1
  Mux/1 -> ICE/1
  Power/1 -> wt (EM1)/1(x), ICE/4, Integrator/1, Pice/1
  avoid division by zero/1 -> Medelvärde/1(In), Fuel power/1
  wice/1 -> Torque limitation/1, Product1/2, wt (ICE)/1(x), "rad/s -> rpm"/1, FuelPower/2(Cols), Efficiency/2(Cols), Power/2
  0.1 sec time constant/1 -> wt (ICE)/2(y), Product1/1, Tice/1, Mux/2, FuelPower/1(Rows), Efficiency/1(Rows), Power/1
  FuelPower/1(Out1) -> Calculate Fuel power directly (w/o idle consumption)/1
  Fuel power/1 -> Calculate Fuel power directly (w/o idle consumption)/2
  Calculate Fuel power directly (w/o idle consumption)/1 -> Fuel Power/1
  Medelvärde/2(Ave) -> EtaICE_AVG/1
  Integrator/1 -> Total_Energy_ICE/1

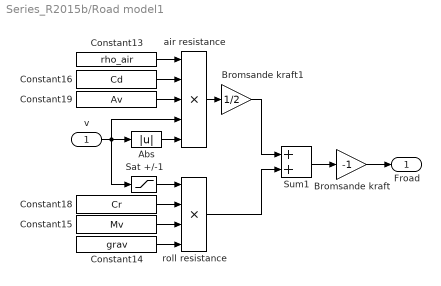
== system Series_R2015b/Road model1 ==
  "v " : Inport
  Abs : Abs  SaturateOnIntegerOverflow=on
  Bromsande kraft : Gain  Gain=-1  SaturateOnIntegerOverflow=on  OutDataTypeStr=Inherit: Same as input  ParamDataTypeStr=Inherit: Same as input
  Bromsande kraft1 : Gain  Gain=1/2  SaturateOnIntegerOverflow=on  OutDataTypeStr=Inherit: Same as input  ParamDataTypeStr=Inherit: Same as input
  Constant13 : Constant  Value=rho_air
  Constant14 : Constant  Value=grav
  Constant15 : Constant  Value=Mv
  Constant16 : Constant  Value=Cd
  Constant18 : Constant  Value=Cr
  Constant19 : Constant  Value=Av
  Sat +/-1 : Saturate  UpperLimit=1  LowerLimit=-1
  Sum1 : Sum  SaturateOnIntegerOverflow=on  InputSameDT=on  OutDataTypeStr=Inherit: Same as first input
  air resistance : Product  Inputs=5  SaturateOnIntegerOverflow=on  InputSameDT=on  OutDataTypeStr=Inherit: Same as first input
  roll resistance : Product  Inputs=4  SaturateOnIntegerOverflow=on  InputSameDT=on  OutDataTypeStr=Inherit: Same as first input
  Froad : Outport  InitialOutput=0
  wires:
  air resistance/1 -> Bromsande kraft1/1
  Bromsande kraft/1 -> Froad/1
  Bromsande kraft1/1 -> Sum1/1
  roll resistance/1 -> Sum1/2
  Sum1/1 -> Bromsande kraft/1
  Constant13/1 -> air resistance/1
  Constant16/1 -> air resistance/2
  Constant19/1 -> air resistance/3
  "v "/1 -> air resistance/4, Sat +/-1/1, Abs/1
  Constant18/1 -> roll resistance/2
  Constant15/1 -> roll resistance/3
  Constant14/1 -> roll resistance/4
  Sat +/-1/1 -> roll resistance/1
  Abs/1 -> air resistance/5

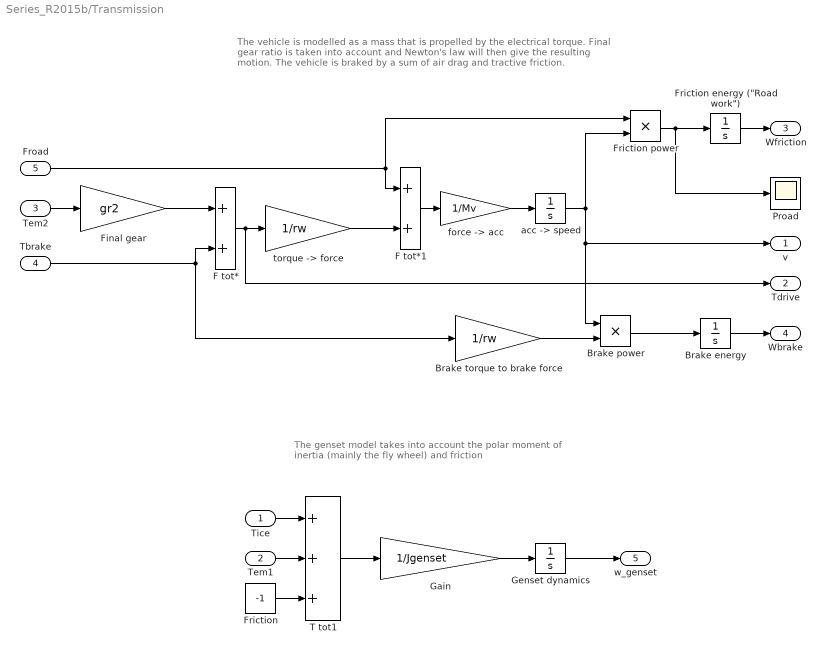
== system Series_R2015b/Transmission ==
  note: The vehicle is modelled as a mass that is propelled by the electrical torque.
      | Final gear ratio is taken into account and Newton's law will then
      | give the resulting motion.
      | The vehicle is braked by a sum of air drag and tractive friction.
  note: The genset model takes into account the polar moment
      | of inertia (mainly the fly wheel) and friction
  Tice : Inport
  Tem1 : Inport  Port=2
  Tem2 : Inport  Port=3
  Tbrake : Inport  Port=4
  Froad : Inport  Port=5
  Brake energy : Integrator
  Brake power : Product  SaturateOnIntegerOverflow=on  InputSameDT=on  OutDataTypeStr=Inherit: Same as first input
  Brake torque to brake force : Gain  Gain=1/rw  SaturateOnIntegerOverflow=on  OutDataTypeStr=Inherit: Same as input  ParamDataTypeStr=Inherit: Same as input
  F tot* : Sum  SaturateOnIntegerOverflow=on  InputSameDT=on  OutDataTypeStr=Inherit: Same as first input
  F tot*1 : Sum  SaturateOnIntegerOverflow=on  InputSameDT=on  OutDataTypeStr=Inherit: Same as first input
  Final gear : Gain  Gain=gr2  SaturateOnIntegerOverflow=on  OutDataTypeStr=Inherit: Same as input  ParamDataTypeStr=Inherit: Same as input
  Friction : Constant  Value=-1
  "Friction energy (\"Road work\")" : Integrator
  Friction power : Product  SaturateOnIntegerOverflow=on  InputSameDT=on  OutDataTypeStr=Inherit: Same as first input
  Gain : Gain  Gain=1/Jgenset  SaturateOnIntegerOverflow=on  OutDataTypeStr=Inherit: Same as input  ParamDataTypeStr=Inherit: Same as input
  Genset dynamics : Integrator
  Proad : Scope
  T tot1 : Sum  Inputs=+++  SaturateOnIntegerOverflow=on  InputSameDT=on  OutDataTypeStr=Inherit: Same as first input
  "acc -> speed" : Integrator
  "force -> acc" : Gain  Gain=1/Mv  SaturateOnIntegerOverflow=on  OutDataTypeStr=Inherit: Same as input  ParamDataTypeStr=Inherit: Same as input
  "torque -> force" : Gain  Gain=1/rw  SaturateOnIntegerOverflow=on  OutDataTypeStr=Inherit: Same as input  ParamDataTypeStr=Inherit: Same as input
  v : Outport  InitialOutput=0
  Tdrive : Outport  Port=2  InitialOutput=0
  Wfriction : Outport  Port=3  InitialOutput=0
  Wbrake : Outport  Port=4  InitialOutput=0
  w_genset : Outport  Port=5  InitialOutput=0
  wires:
  "force -> acc"/1 -> "acc -> speed"/1
  Tem2/1 -> Final gear/1
  "acc -> speed"/1 -> Brake power/1, v/1, Friction power/2
  F tot*/1 -> "torque -> force"/1, Tdrive/1
  Tbrake/1 -> F tot*/2, Brake torque to brake force/1
  "torque -> force"/1 -> F tot*1/2
  F tot*1/1 -> "force -> acc"/1
  Froad/1 -> Friction power/1, F tot*1/1
  Brake torque to brake force/1 -> Brake power/2
  Brake power/1 -> Brake energy/1
  Friction power/1 -> "Friction energy (\"Road work\")"/1, Proad/1
  "Friction energy (\"Road work\")"/1 -> Wfriction/1
  Brake energy/1 -> Wbrake/1
  Genset dynamics/1 -> w_genset/1
  Tice/1 -> T tot1/1
  Tem1/1 -> T tot1/2
  T tot1/1 -> Gain/1
  Gain/1 -> Genset dynamics/1
  Friction/1 -> T tot1/3
  Final gear/1 -> F tot*/1

== system Series_R2015b/Battery/Chemical Power ==
  Pterm : Inport
  Look-Up Table : Lookup  InputValues=Pbatt  Table=EtaBATT  SaturateOnIntegerOverflow=on
  P/ n : Product  Inputs=**  SaturateOnIntegerOverflow=on  InputSameDT=on  OutDataTypeStr=Inherit: Same as first input
  Saturation : Saturate  UpperLimit=max(Pbatt)  LowerLimit=min(Pbatt)
  Pcharge : Outport  InitialOutput=0
  eta : Outport  Port=2  InitialOutput=0
  wires:
  Pterm/1 -> P/ n/1, Saturation/1
  Saturation/1 -> Look-Up Table/1
  P/ n/1 -> Pcharge/1
  Look-Up Table/1 -> P/ n/2, eta/1

== system Series_R2015b/Battery/Subsystem ==
  "Pcharge " : Inport
  Constant : Constant  Value=SOC_batt_ref_value/100*Wbatt
  Gain3 : Gain  Gain=100/Wbatt  SaturateOnIntegerOverflow=on  OutDataTypeStr=Inherit: Same as input  ParamDataTypeStr=Inherit: Same as input
  Ptrm1 : Sum  Inputs=+-  SaturateOnIntegerOverflow=on  InputSameDT=on  OutDataTypeStr=Inherit: Same as first input
  W batt starts at SOC_batt_ref_value : Integrator  InitialCondition=SOC_batt_ref_value/100*Wbatt  LimitOutput=on  LowerSaturationLimit=0
  W batt in [%] : Outport
  DeltaWbatt in [Ws] : Outport  Port=2
  wires:
  W batt starts at SOC_batt_ref_value/1 -> Gain3/1, Ptrm1/1
  Gain3/1 -> W batt in [%]/1
  Constant/1 -> Ptrm1/2
  Ptrm1/1 -> DeltaWbatt in [Ws]/1
  "Pcharge "/1 -> W batt starts at SOC_batt_ref_value/1

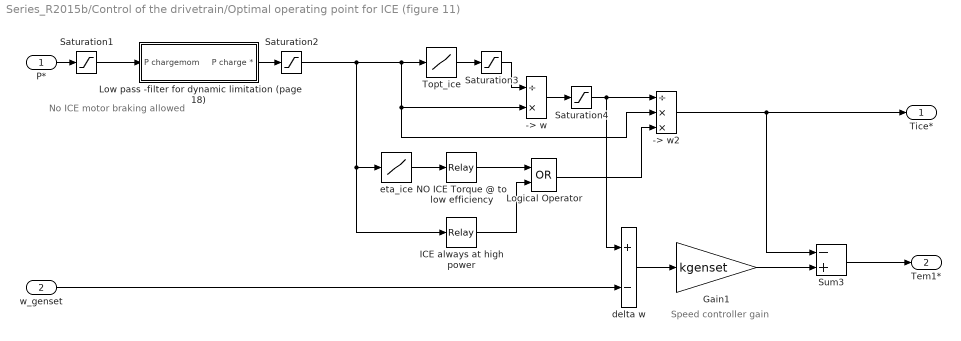
== system Series_R2015b/Control of the drivetrain/Optimal operating point for ICE (figure 11) ==
  note: No ICE motor
      | braking allowed
  note: Speed controller gain
  P* : Inport
  w_genset : Inport  Port=2
  -> w : Product  Inputs=/*  SaturateOnIntegerOverflow=on  InputSameDT=on  OutDataTypeStr=Inherit: Same as first input
  -> w2 : Product  Inputs=/**  SaturateOnIntegerOverflow=on  InputSameDT=on  OutDataTypeStr=Inherit: Same as first input
  Gain1 : Gain  Gain=kgenset  SaturateOnIntegerOverflow=on  OutDataTypeStr=Inherit: Same as input  ParamDataTypeStr=Inherit: Same as input
  ICE always at high power : Relay  OnSwitchValue=Pice_max/1.8*1.1  OffSwitchValue=Pice_max/1.8*0.9
  Logical Operator : Logic  Operator=OR  AllPortsSameDT=off
  Low pass -filter for dynamic limitation (page 18) : Subsystem
  NO ICE Torque @ to low efficiency : Relay  OnSwitchValue=0.28  OffSwitchValue=0.25
  Saturation1 : Saturate  UpperLimit=inf  LowerLimit=eps
  Saturation2 : Saturate  UpperLimit=Pice_max  LowerLimit=eps
  Saturation3 : Saturate  UpperLimit=Tice_max  LowerLimit=eps
  Saturation4 : Saturate  UpperLimit=wice_max  LowerLimit=wice_min
  Sum3 : Sum  Inputs=-+  SaturateOnIntegerOverflow=on  InputSameDT=on  OutDataTypeStr=Inherit: Same as first input
  Topt_ice : Lookup  InputValues=PtoT(:,1)  Table=PtoT(:,2)  SaturateOnIntegerOverflow=on
  delta w : Sum  Inputs=+-  SaturateOnIntegerOverflow=on  InputSameDT=on  OutDataTypeStr=Inherit: Same as first input
  eta_ice : Lookup  InputValues=PtoT(:,1)  Table=PtoT(:,3)  SaturateOnIntegerOverflow=on
  Tice* : Outport  InitialOutput=0
  Tem1* : Outport  Port=2  InitialOutput=0
  wires:
  P*/1 -> Saturation1/1
  -> w/1 -> Saturation4/1
  Topt_ice/1 -> Saturation3/1
  Low pass -filter for dynamic limitation (page 18)/1(P charge *) -> Saturation2/1
  Saturation1/1 -> Low pass -filter for dynamic limitation (page 18)/1(P chargemom)
  Saturation3/1 -> -> w/1
  delta w/1 -> Gain1/1
  w_genset/1 -> delta w/2
  Saturation4/1 -> -> w2/1, delta w/1
  Gain1/1 -> Sum3/2
  Saturation2/1 -> ICE always at high power/1, eta_ice/1, Topt_ice/1, -> w/2, -> w2/2
  eta_ice/1 -> NO ICE Torque @ to low efficiency/1
  NO ICE Torque @ to low efficiency/1 -> Logical Operator/1
  ICE always at high power/1 -> Logical Operator/2
  Logical Operator/1 -> -> w2/3
  -> w2/1 -> Sum3/1, Tice*/1
  Sum3/1 -> Tem1*/1

== system Series_R2015b/Control of the drivetrain/SOC controller (Eq. 3-9) ==
  SOC : Inport
  SOC controller gain : Gain  Gain=ksoc  OutDataTypeStr=Inherit: Same as input  ParamDataTypeStr=Inherit: Same as input
  SOC* : Constant  Value=SOC_batt_ref_value
  Sum1 : Sum  Inputs=-+  SaturateOnIntegerOverflow=on  InputSameDT=on  OutDataTypeStr=Inherit: Same as first input
  P charge * : Outport  InitialOutput=0
  wires:
  SOC*/1 -> Sum1/2
  Sum1/1 -> SOC controller gain/1
  SOC/1 -> Sum1/1
  SOC controller gain/1 -> P charge */1

== system Series_R2015b/EM1 (Generator)/Medelvärde ==
  note: Denna del "mäter" tiden då motorn
      | är till, d.v.s. då verkningsgraden är
      | större än 1 %. Om den är 5 % antas
      | motorn stå still.
  In : Inport
  Integral : Integrator
  Integral1 : Integrator  InitialCondition=1  LimitOutput=on  LowerSaturationLimit=1
  Medelv : Product  Inputs=*/  SaturateOnIntegerOverflow=on  InputSameDT=on  OutDataTypeStr=Inherit: Same as first input
  Medelv1 : Product  Inputs=**  SaturateOnIntegerOverflow=on  InputSameDT=on  OutDataTypeStr=Inherit: Same as first input
  Relay : Relay  OnSwitchValue=0.05  OffSwitchValue=0.04
  Scope : Scope  NumInputPorts=3
  Ave : Outport
  wires:
  Integral1/1 -> Medelv/2
  Integral/1 -> Medelv/1
  In/1 -> Scope/2, Relay/1, Medelv1/1
  Relay/1 -> Scope/1, Integral1/1, Medelv1/2
  Medelv/1 -> Ave/1, Scope/3
  Medelv1/1 -> Integral/1

== system Series_R2015b/EM1 (Generator)/Subsystem ==
  T : Inport
  w : Inport  Port=2
  Abs2 : Abs  SaturateOnIntegerOverflow=on
  Constant : Constant  Value=eps
  EM torque1 : Product  Inputs=/*  SaturateOnIntegerOverflow=on  InputSameDT=on  OutDataTypeStr=Inherit: Same as first input
  T*w_ice : Product  Inputs=**  SaturateOnIntegerOverflow=on  InputSameDT=on  OutDataTypeStr=Inherit: Same as first input
  maxP : Saturate  UpperLimit=Pmax  LowerLimit=-Pmax
  maxT : Saturate  UpperLimit=Tmax  LowerLimit=-Tmax
  not div by 0 : Sum  SaturateOnIntegerOverflow=on  InputSameDT=on  OutDataTypeStr=Inherit: Same as first input
  Tlim : Outport
  wires:
  w/1 -> Abs2/1
  T/1 -> T*w_ice/2
  T*w_ice/1 -> maxP/1
  maxP/1 -> EM torque1/2
  maxT/1 -> Tlim/1
  EM torque1/1 -> maxT/1
  Constant/1 -> not div by 0/1
  not div by 0/1 -> EM torque1/1
  Abs2/1 -> T*w_ice/1, not div by 0/2

== system Series_R2015b/EM1 (Generator)/wt (EM1) ==
  x : Inport
  y : Inport  Port=2
  Mux : Mux  Inputs=2
  sfunxy : S-Function  DisableCoverage=on  FunctionName=sfunxy  Parameters=[xmin xmax ymin ymax], st  SFunctionDeploymentMode=off  EnableBusSupport=off
  wires:
  y/1 -> Mux/2
  x/1 -> Mux/1
  Mux/1 -> sfunxy/1

== system Series_R2015b/EM2 (Traction Motor)/Medelvärde ==
  note: Denna del "mäter" tiden då motorn
      | är till, d.v.s. då verkningsgraden är
      | större än 1 %. Om den är 5 % antas
      | motorn stå still.
  In : Inport
  Integral : Integrator
  Integral1 : Integrator  InitialCondition=1  LimitOutput=on  LowerSaturationLimit=1
  Medelv : Product  Inputs=*/  SaturateOnIntegerOverflow=on  InputSameDT=on  OutDataTypeStr=Inherit: Same as first input
  Medelv1 : Product  Inputs=**  SaturateOnIntegerOverflow=on  InputSameDT=on  OutDataTypeStr=Inherit: Same as first input
  Relay : Relay  OnSwitchValue=0.05  OffSwitchValue=0.04
  Scope : Scope  NumInputPorts=3
  Ave : Outport
  wires:
  Integral1/1 -> Medelv/2
  Integral/1 -> Medelv/1
  In/1 -> Scope/2, Relay/1, Medelv1/1
  Relay/1 -> Scope/1, Integral1/1, Medelv1/2
  Medelv/1 -> Ave/1, Scope/3
  Medelv1/1 -> Integral/1

== system Series_R2015b/EM2 (Traction Motor)/Subsystem ==
  T : Inport
  w : Inport  Port=2
  Abs2 : Abs  SaturateOnIntegerOverflow=on
  EM torque1 : Product  Inputs=/*  SaturateOnIntegerOverflow=on  InputSameDT=on  OutDataTypeStr=Inherit: Same as first input
  T*w_ice : Product  Inputs=**  SaturateOnIntegerOverflow=on  InputSameDT=on  OutDataTypeStr=Inherit: Same as first input
  eps : Saturate  UpperLimit=inf  LowerLimit=eps
  maxP : Saturate  UpperLimit=Pmax  LowerLimit=-Pmax
  maxT : Saturate  UpperLimit=Tmax  LowerLimit=-Tmax
  Tlim : Outport
  wires:
  w/1 -> Abs2/1
  T/1 -> T*w_ice/2
  T*w_ice/1 -> maxP/1
  maxP/1 -> EM torque1/2
  maxT/1 -> Tlim/1
  EM torque1/1 -> maxT/1
  eps/1 -> T*w_ice/1, EM torque1/1
  Abs2/1 -> eps/1

== system Series_R2015b/EM2 (Traction Motor)/wt (EM2) ==
  x : Inport
  y : Inport  Port=2
  Mux : Mux  Inputs=2
  sfunxy : S-Function  DisableCoverage=on  FunctionName=sfunxy  Parameters=[xmin xmax ymin ymax], st  SFunctionDeploymentMode=off  EnableBusSupport=off
  wires:
  y/1 -> Mux/2
  x/1 -> Mux/1
  Mux/1 -> sfunxy/1

== system Series_R2015b/ICE-model/Efficiency ==
  Rows : Inport
  Cols : Inport  Port=2
  Look-Up Table (2-D) : Lookup2D  RowIndex=x  ColumnIndex=y  Table=t  SaturateOnIntegerOverflow=on  InputSameDT=on
  Out1 : Outport
  wires:
  Rows/1 -> Look-Up Table (2-D)/1
  Cols/1 -> Look-Up Table (2-D)/2
  Look-Up Table (2-D)/1 -> Out1/1

== system Series_R2015b/ICE-model/FuelPower ==
  Rows : Inport
  Cols : Inport  Port=2
  Look-Up Table (2-D) : Lookup2D  RowIndex=x  ColumnIndex=y  Table=t  SaturateOnIntegerOverflow=on  InputSameDT=on
  Out1 : Outport
  wires:
  Look-Up Table (2-D)/1 -> Out1/1
  Cols/1 -> Look-Up Table (2-D)/2
  Rows/1 -> Look-Up Table (2-D)/1

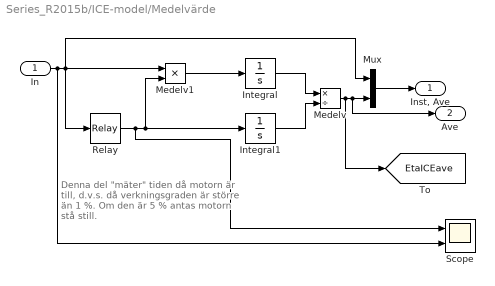
== system Series_R2015b/ICE-model/Medelvärde ==
  note: Denna del "mäter" tiden då motorn
      | är till, d.v.s. då verkningsgraden är
      | större än 1 %. Om den är 5 % antas
      | motorn stå still.
  In : Inport
  Integral : Integrator
  Integral1 : Integrator  InitialCondition=1  LimitOutput=on  LowerSaturationLimit=1
  Medelv : Product  Inputs=*/  SaturateOnIntegerOverflow=on  InputSameDT=on  OutDataTypeStr=Inherit: Same as first input
  Medelv1 : Product  Inputs=**  SaturateOnIntegerOverflow=on  InputSameDT=on  OutDataTypeStr=Inherit: Same as first input
  Mux : Mux  Inputs=2
  Relay : Relay  OnSwitchValue=0.05  OffSwitchValue=0.04
  Scope : Scope  NumInputPorts=2
  "Inst, Ave" : Outport
  Ave : Outport  Port=2
  tag scope: EtaICEave=global
  wires:
  Integral1/1 -> Medelv/2
  Integral/1 -> Medelv/1
  In/1 -> Scope/2, Relay/1, Mux/1, Medelv1/1
  Relay/1 -> Scope/1, Integral1/1, Medelv1/2
  Medelv/1 -> Ave/1, Mux/2, [EtaICEave]
  Mux/1 -> "Inst, Ave"/1
  Medelv1/1 -> Integral/1

== system Series_R2015b/ICE-model/wt (EM1) ==
  x : Inport
  y : Inport  Port=2
  Mux : Mux  Inputs=2
  sfunxy : S-Function  DisableCoverage=on  FunctionName=sfunxy  Parameters=[xmin xmax ymin ymax], st  SFunctionDeploymentMode=off  EnableBusSupport=off
  wires:
  y/1 -> Mux/2
  x/1 -> Mux/1
  Mux/1 -> sfunxy/1

== system Series_R2015b/ICE-model/wt (ICE) ==
  x : Inport
  y : Inport  Port=2
  Mux : Mux  Inputs=2
  sfunxy : S-Function  DisableCoverage=on  FunctionName=sfunxy  Parameters=[xmin xmax ymin ymax], st  SFunctionDeploymentMode=off  EnableBusSupport=off
  wires:
  y/1 -> Mux/2
  x/1 -> Mux/1
  Mux/1 -> sfunxy/1

== system Series_R2015b/Control of the drivetrain/Optimal operating point for ICE (figure 11)/Low pass -filter for dynamic limitation (page 18) ==
  P chargemom : Inport
  Gain2 : Gain  Gain=1/(Tau_charge)  SaturateOnIntegerOverflow=on  OutDataTypeStr=Inherit: Same as input  ParamDataTypeStr=Inherit: Same as input
  Sum3 : Sum  Inputs=+-  SaturateOnIntegerOverflow=on  InputSameDT=on  OutDataTypeStr=Inherit: Same as first input
  Wbatt : Integrator  UpperSaturationLimit=Pice_max_parallel  LowerSaturationLimit=0
  P charge * : Outport  InitialOutput=0
  wires:
  P chargemom/1 -> Sum3/1
  Sum3/1 -> Gain2/1
  Gain2/1 -> Wbatt/1
  Wbatt/1 -> Sum3/2, P charge */1
